simulink model "semibatchreactor"  (R2018a)
settings: Solver=VariableStepAuto  StartTime=0.0  StopTime=500  RelTol=1e-3
settings Model: Creator=kudva  LastModifiedBy=kudva

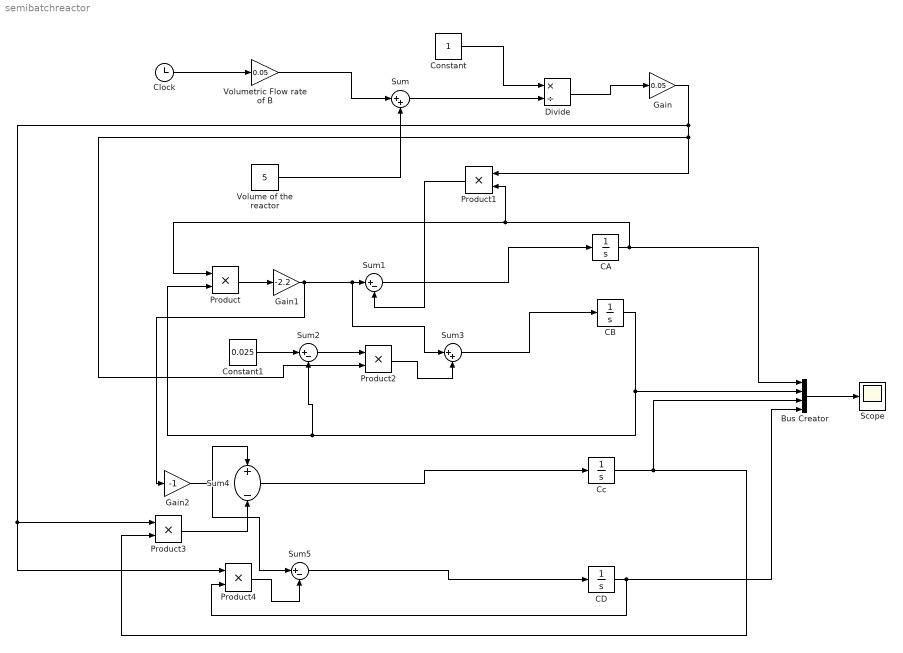
== system semibatchreactor ==
  Bus Creator : BusCreator  Inputs=4
  "CA " : Integrator  InitialCondition=0.05
  CB : Integrator
  CD : Integrator
  Cc : Integrator
  Clock : Clock
  Constant : Constant
  Constant1 : Constant  Value=0.025
  Divide : Product  Inputs=*/
  Gain : Gain  Gain=0.05
  Gain1 : Gain  Gain=-2.2
  Gain2 : Gain  Gain=-1
  Product{,1..4} (5 alike) : Product
  Scope : Scope
  Sum : Sum  Inputs=|++
  Sum1 : Sum  Inputs=|+-
  Sum2 : Sum  Inputs=|+-
  Sum3 : Sum  Inputs=|++
  Sum4 : Sum  Inputs=+-
  Sum5 : Sum  Inputs=|+-
  "Volume of the reactor " : Constant  Value=5
  Volumetric Flow rate of B : Gain  Gain=0.05
  wires:
  "Volume of the reactor "/1 -> Sum/2
  Volumetric Flow rate of B/1 -> Sum/1
  Clock/1 -> Volumetric Flow rate of B/1
  Sum/1 -> Divide/2
  Constant/1 -> Divide/1
  Divide/1 -> Gain/1
  Product/1 -> Gain1/1
  CB/1 -> Bus Creator/2, Sum2/2, Product/2
  "CA "/1 -> Bus Creator/1, Product1/2, Product/1
  Gain/1 -> Product1/1, Product2/2, Product3/1, Product4/1
  Product1/1 -> Sum1/2
  Gain1/1 -> Gain2/1, Sum3/1, Sum1/1
  Sum1/1 -> "CA "/1
  Constant1/1 -> Sum2/1
  Sum2/1 -> Product2/1
  Product2/1 -> Sum3/2
  Sum3/1 -> CB/1
  Gain2/1 -> Sum5/1, Sum4/1
  Cc/1 -> Product3/2, Bus Creator/3
  Product3/1 -> Sum4/2
  Sum4/1 -> Cc/1
  CD/1 -> Bus Creator/4, Product4/2
  Product4/1 -> Sum5/2
  Sum5/1 -> CD/1
  Bus Creator/1 -> Scope/1
